simulink subsystem "DCMotorModelSimple"  (R2023b)
settings: Solver=VariableStepAuto  StartTime=0.0  StopTime=10.0  RelTol=1e-3
model mask{T_max=0.000953, w_max=1570.79632679, V_max=6}
values from neighbouring files (symbols this model uses):
  B = 20    [quaternionTest.m]
undefined symbols (not defined in the file or in its folder): J, Kt
libraries: slpidlib x1
settings Model: Creator=andrea  LastModifiedBy=andrea

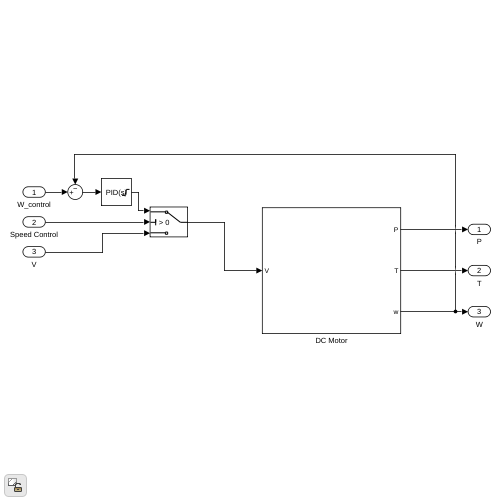
[thumbnail: Simulink's stored preview of the top-level diagram]
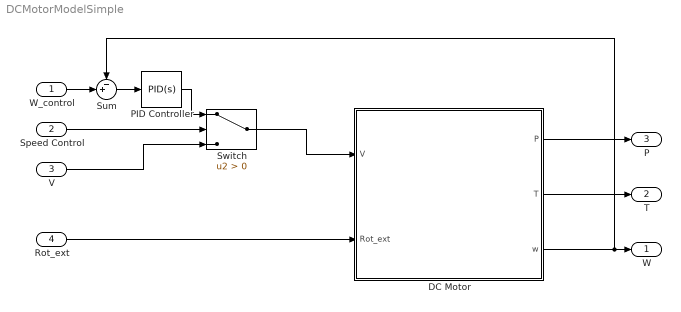
== system DCMotorModelSimple ==
  W_control : Inport
  Speed Control : Inport  Port=2
  V : Inport  Port=3
  Rot_ext : Inport  Port=4
  DC Motor : Subsystem
  PID Controller : slpidlib/PID Controller  Controller=PID  Form=Parallel  TimeDomain=Continuous-time  UseExternalTs=off  SampleTime=-1  IntegratorMethod=Forward Euler  FilterMethod=Forward Euler  ControllerParametersSource=internal  P=0.0135694485712718  I=0.254571726895349  UseKiTs=off  D=0  N=61.146147680322  UseFilter=on  TunerSelectOption=Transfer Function Based (PID Tuner App)  InitialConditionSource=internal  InitialConditionForIntegrator=0  InitialConditionForFilter=0  DifferentiatorICPrevScaledInput=0  ExternalReset=none  TrackingMode=off  Kt=1  LimitOutput=on  SatLimitsSource=internal  UpperSaturationLimit=6  LowerSaturationLimit=-6  LinearizeAsGain=on  AntiWindupMode=clamping  Kb=1  LimitIntegrator=on  UpperIntegratorSaturationLimit=6  LowerIntegratorSaturationLimit=-6  POutMin=[]  POutMax=[]  IOutMin=[]  IOutMax=[]  DOutMin=[]  DOutMax=[]  NOutMin=[]  NOutMax=[]  SumOutMin=[]  SumOutMax=[]  SaturationOutMin=[]  SaturationOutMax=[]  PParamMin=[]  PParamMax=[]  IParamMin=[]  IParamMax=[]  DParamMin=[]  DParamMax=[]  NParamMin=[]  NParamMax=[]  KbParamMin=[]  KbParamMax=[]  KtParamMin=[]  KtParamMax=[]  KbOutMin=[]  KbOutMax=[]  KtOutMin=[]  KtOutMax=[]  IntegratorOutMin=[]  IntegratorOutMax=[]  FilterOutMin=[]  FilterOutMax=[]  SumI1OutMin=[]  SumI1OutMax=[]  SumI2OutMin=[]  SumI2OutMax=[]  SumI3OutMin=[]  SumI3OutMax=[]  SumI4OutMin=[]  SumI4OutMax=[]  SumDOutMin=[]  SumDOutMax=[]  DifferentiatorOutMin=[]  DifferentiatorOutMax=[]  FilterDiffOutCoefMin=[]  FilterDiffOutCoefMax=[]  ReciprocalOutMin=[]  ReciprocalOutMax=[]  SumDenOutMin=[]  SumDenOutMax=[]  SumNumOutMin=[]  SumNumOutMax=[]  DivideOutMin=[]  DivideOutMax=[]  UdiffTsProdOutMin=[]  UdiffTsProdOutMax=[]  NTsProdOutMin=[]  NTsProdOutMax=[]  UintegralTsProdOutMin=[]  UintegralTsProdOutMax=[]  UngainTsProdOutMin=[]  UngainTsProdOutMax=[]  ClampingZeroOutDataTypeStr=Inherit: Inherit via back propagation  ClampingZeroOutMin=[]  ClampingZeroOutMax=[]  FilterDenConstantOutDataTypeStr=Inherit: Inherit via back propagation  FilterDenConstantOutMin=[]  FilterDenConstantOutMax=[]  PCopyOutDataTypeStr=Inherit: Inherit via back propagation  PCopyOutMin=[]  PCopyOutMax=[]  NCopyOutDataTypeStr=Inherit: Inherit via back propagation  NCopyOutMin=[]  NCopyOutMax=[]  IntegratorContinuousStateAttributes=''  IntegratorStateMustResolveToSignalObject=off  IntegratorRTWStateStorageClass=Auto  FilterContinuousStateAttributes=''  FilterStateMustResolveToSignalObject=off  FilterRTWStateStorageClass=Auto  ParallelPVariant=InternalParameters  IdealPVariant=Disabled  IVariant=InternalParameters  DVariant=InternalParameters  IntegratorVariant=Continuous  SatVariant=Enabled  AWVariant=ContClampingParallel  PCopyVariant=Disabled  TRVariant=Disabled  FdbkBlocksVariant=Forward  IdealPFdbkVariant=Disabled  SatFdbkVariant=Disabled  DerivativeFilterVariant=ContFilter  NVariant=InternalParameters  NCopyVariant=Disabled  FilterICVariant=InternalICsFilter  IntegratorICVariant=InternalICs  ExternalResetVariant=Disabled  TRSumVariant=Passthrough  SumFdbkVariant=Disabled  SumVariant=Sum_PID  TsampFilterVariant=InternalTs  TsampNgainVariant=Passthrough  TsampIntegralVariant=Disabled_SignalSpec  ExternalSaturationOutDataTypeStr=Inherit: Same as second input
  Sum : Sum  Inputs=-+|
  Switch : Switch  Criteria=u2 > Threshold  SaturateOnIntegerOverflow=off  InputSameDT=off
  W : Outport
  T : Outport  Port=2
  P : Outport  Port=3
  wires:
  W_control/1 -> Sum/2
  DC Motor/2(T) -> T/1
  Speed Control/1 -> Switch/2
  PID Controller/1 -> Switch/1
  DC Motor/3(w) -> W/1, Sum/1
  V/1 -> Switch/3
  Switch/1 -> DC Motor/1(V)
  Sum/1 -> PID Controller/1
  DC Motor/1(P) -> P/1
  Rot_ext/1 -> DC Motor/2(Rot_ext)

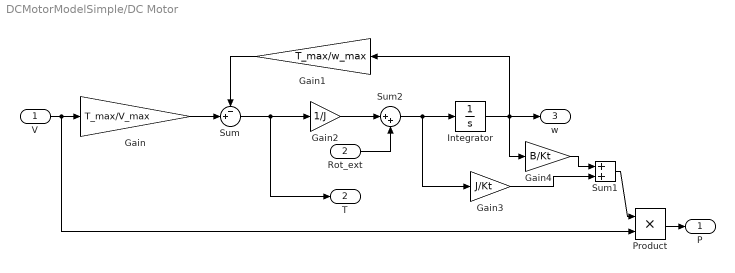
== system DCMotorModelSimple/DC Motor ==
  V : Inport
  Rot_ext : Inport  Port=2
  Gain : Gain  Gain=T_max/V_max
  Gain1 : Gain  Gain=T_max/w_max
  Gain2 : Gain  Gain=1/J
  Gain3 : Gain  Gain=J/Kt
  Gain4 : Gain  Gain=B/Kt
  Integrator : Integrator
  Product : Product
  Sum : Sum  Inputs=-+|
  Sum1 : Sum
  Sum2 : Sum  Inputs=|++
  P : Outport
  T : Outport  Port=2
  w : Outport  Port=3
  wires:
  Gain2/1 -> Sum2/1
  Sum2/1 -> Integrator/1, Gain3/1
  Sum/1 -> T/1, Gain2/1
  Rot_ext/1 -> Sum2/2
  Product/1 -> P/1
  Sum1/1 -> Product/1
  Gain3/1 -> Sum1/2
  Gain4/1 -> Sum1/1
  Integrator/1 -> Gain1/1, w/1, Gain4/1
  Gain1/1 -> Sum/1
  Gain/1 -> Sum/2
  V/1 -> Gain/1, Product/2
